simulink model "kopter_se_zavazim_LQR"  (R2024b)
settings: Solver=FixedStepAuto  StartTime=0.0  StopTime=30  FixedStep=0.01  RelTol=1e-3
values from neighbouring files (symbols this model uses):
  b_moment = 5.4e-6    (= 5.4e-06)    [parametry_kopter_se_zavazim.m]
  d = 1    [parametry_kopter_se_zavazim.m]
  g = 9.81    [parametry_kopter_se_zavazim.m]
  Ip = m*d^2    (= 1)    [parametry_kopter_se_zavazim.m]
  Ixx = 0.0222    [parametry_kopter_se_zavazim.m]
  Iyy = 0.0222    [parametry_kopter_se_zavazim.m]
  Izz = 0.0429    [parametry_kopter_se_zavazim.m]
  k_thrust = 2.3e-3    (= 0.0023)    [parametry_kopter_se_zavazim.m]
  ki_lqr = K_ex_lqr(:, 17:20)    [odvozeni_stavova_regulace_OTHER_ANGLES.m]
  kimot_lqr = Kmot_ex_lqr(:, 17:20)    [odvozeni_stavova_regulace_OTHER_ANGLES.m]
  kp_lqr = K_ex_lqr(:, 1:16)    [odvozeni_stavova_regulace_OTHER_ANGLES.m]
  kpmot_lqr = Kmot_ex_lqr(:, 1:16)    [odvozeni_stavova_regulace_OTHER_ANGLES.m]
  l = 0.2051    [parametry_kopter_se_zavazim.m]
  L_observer = place(Ac', Cc', poles_obs)'    [odvozeni_stavova_regulace_OTHER_ANGLES.m]
  M = 2    [parametry_kopter_se_zavazim.m]
  m = 1    [parametry_kopter_se_zavazim.m]
  Us_p = [(M+m)*g; 0; 0; 0]    [parametry_kopter_se_zavazim.m]
  Xinit_ss = [Xinit_matrix; [0 0 0 0 0 0 0 0]']    [parametry_kopter_se_zavazim.m]
  Xs_p = [0;0;0; 0;0;0; 0;0; 0;0;0; 0;0;0; 0;0]    [parametry_kopter_se_zavazim.m]
undefined symbols (not defined in the file or in its folder): L
libraries: simulink_extras x10
(part 3 of 3)

== matlab function kopter_se_zavazim_LQR/Nelinearni State-Space (se zavazim)_other_angles/A ==
  data: roll input; A output; pitch input; yaw input; alpha input; beta input; droll input; dpitch input; dyaw input; dalpha input; dbeta input; Ixx parameter; Iyy parameter; Izz parameter; M parameter; Ip parameter; d parameter; m parameter
function A = fcn(roll, pitch, yaw, alpha, beta, droll, dpitch, dyaw, dalpha, dbeta, Ixx, Iyy, Izz, M, Ip, d, m)
% Matice dynamiky A

phi_t = roll;
theta_t = pitch;
psi_t = yaw;

alpha_t = alpha;
beta_t = beta;

phi_dot_t = droll;
theta_dot_t = dpitch;
psi_dot_t = dyaw;

alpha_dot_t = dalpha;
beta_dot_t = dbeta;

A = [ 
0, 0, 0, 0, 0, 0, 0, 0, 1, 0, 0,                                                                                                                                                                                                                                                                                                                                                                                                                                                                                                           0,                                                                                                                                                                                                                                                                                                                                                                                                                                                                                                                                                                                                                                                                                                                              0,                                                                                                                                                                                            0,                                                          0,                                                  0;
0, 0, 0, 0, 0, 0, 0, 0, 0, 1, 0,                                                                                                                                                                                                                                                                                                                                                                                                                                                                                                           0,                                                                                                                                                                                                                                                                                                                                                                                                                                                                                                                                                                                                                                                                                                                              0,                                                                                                                                                                                            0,                                                          0,                                                  0;
0, 0, 0, 0, 0, 0, 0, 0, 0, 0, 1,                                                                                                                                                                                                                                                                                                                                                                                                                                                                                                           0,                                                                                                                                                                                                                                                                                                                                                                                                                                                                                                                                                                                                                                                                                                                              0,                                                                                                                                                                                            0,                                                          0,                                                  0;
0, 0, 0, 0, 0, 0, 0, 0, 0, 0, 0,                                                                                                                                                                                                                                                                                                                                                                                                                                                                                                           1,                                                                                                                                                                                                                                                                                                                                                                                                                                                                                                                                                                                                                                                                                                                              0,                                                                                                                                                                                            0,                                                          0,                                                  0;
0, 0, 0, 0, 0, 0, 0, 0, 0, 0, 0,                                                                                                                                                                                                                                                                                                                                                                                                                                                                                                           0,                                                                                                                                                                                                                                                                                                                                                                                                                                                                                                                                                                                                                                                                                                                              1,                                                                                                                                                                                            0,                                                          0,                                                  0;
0, 0, 0, 0, 0, 0, 0, 0, 0, 0, 0,                                                                                                                                                                                                                                                                                                                                                                                                                                                                                                           0,                                                                                                                                                                                                                                                                                                                                                                                                                                                                                                                                                                                                                                                                                                                              0,                                                                                                                                                                                            1,                                                          0,                                                  0;
0, 0, 0, 0, 0, 0, 0, 0, 0, 0, 0,                                                                                                                                                                                                                                                                                                                                                                                                                                                                                                           0,                                                                                                                                                                                                                                                                                                                                                                                                                                                                                                                                                                                                                                                                                                                              0,                                                                                                                                                                                            0,                                                          1,                                                  0;
0, 0, 0, 0, 0, 0, 0, 0, 0, 0, 0,                                                                                                                                                                                                                                                                                                                                                                                                                                                                                                           0,                                                                                                                                                                                                                                                                                                                                                                                                                                                                                                                                                                                                                                                                                                                              0,                                                                                                                                                                                            0,                                                          0,                                                  1;
0, 0, 0, 0, 0, 0, 0, 0, 0, 0, 0,                                                                                                                                                                                                                                                                                                                                                                                                                                                                                                           0,                                                                                                                                                                                                                                                                                                                                                                                                                                                                                                                                                                                                                                                                                                                              0,                                                                                                                                                                                            0,       (alpha_dot_t*d*m*cos(beta_t)^3*sin(alpha_t))/(M + m),  (beta_dot_t*d*m*cos(beta_t)*sin(alpha_t))/(M + m);
0, 0, 0, 0, 0, 0, 0, 0, 0, 0, 0,                                                                                                                                                                                                                                                                                                                                                                                                                                                                                                           0,                                                                                                                                                                                                                                                                                                                                                                                                                                                                                                                                                                                                                                                                                                                              0,                                                                                                                                                                                            0, -(alpha_dot_t*d*m*sin(beta_t)*(sin(beta_t)^2 - 1))/(M + m),               (beta_dot_t*d*m*sin(beta_t))/(M + m);
0, 0, 0, 0, 0, 0, 0, 0, 0, 0, 0,                                                                                                                                                                                                                                                                                                                                                                                                                                                                                                           0,                                                                                                                                                                                                                                                                                                                                                                                                                                                                                                                                                                                                                                                                                                                              0,                                                                                                                                                                                            0,      -(alpha_dot_t*d*m*cos(alpha_t)*cos(beta_t)^3)/(M + m), -(beta_dot_t*d*m*cos(alpha_t)*cos(beta_t))/(M + m);
0, 0, 0, 0, 0, 0, 0, 0, 0, 0, 0,                                       (sin(theta_t)*(Ixx*Izz*theta_dot_t - Izz^2*theta_dot_t + Iyy*Izz*theta_dot_t - Iyy^2*theta_dot_t*cos(phi_t)^2 + Izz^2*theta_dot_t*cos(phi_t)^2 + Ixx*Iyy*theta_dot_t*cos(phi_t)^2 - Ixx*Izz*theta_dot_t*cos(phi_t)^2 - Iyy^2*psi_dot_t*cos(phi_t)*cos(theta_t)*sin(phi_t) + Izz^2*psi_dot_t*cos(phi_t)*cos(theta_t)*sin(phi_t) + Ixx*Iyy*psi_dot_t*cos(phi_t)*cos(theta_t)*sin(phi_t) - Ixx*Izz*psi_dot_t*cos(phi_t)*cos(theta_t)*sin(phi_t)))/(Iyy*Izz*cos(theta_t)), - ((Iyy*Izz + Ixx*Iyy*sin(theta_t)^2 - Iyy*Izz*sin(theta_t)^2 - Ixx*Iyy*sin(phi_t)^2*sin(theta_t)^2 + Ixx*Izz*sin(phi_t)^2*sin(theta_t)^2)*((Izz*theta_dot_t*sin(2*phi_t))/2 - (Iyy*theta_dot_t*sin(2*phi_t))/2 + Ixx*psi_dot_t*cos(theta_t) - Iyy*psi_dot_t*cos(theta_t) + Izz*psi_dot_t*cos(theta_t) + 2*Iyy*psi_dot_t*cos(phi_t)^2*cos(theta_t) - 2*Izz*psi_dot_t*cos(phi_t)^2*cos(theta_t)))/(Ixx*Iyy*Izz*(sin(theta_t)^2 - 1)) - (sin(theta_t)^2*(Iyy - Iyy*sin(phi_t)^2 + Izz*sin(phi_t)^2)*((Iyy*theta_dot_t*sin(2*phi_t))/2 - (Izz*theta_dot_t*sin(2*phi_t))/2 - 2*Ixx*psi_dot_t*cos(theta_t) + 2*Izz*psi_dot_t*cos(phi_t)^2*cos(theta_t) + 2*Iyy*psi_dot_t*cos(theta_t)*sin(phi_t)^2))/(Iyy*Izz*(sin(theta_t)^2 - 1)), (psi_dot_t*sin(2*phi_t)*(Iyy - Izz)*(Ixx^2*cos(2*theta_t) - Ixx^2 + Ixx*Iyy + Ixx*Izz + Iyy*Izz - Ixx*Iyy*cos(2*theta_t) - Ixx*Izz*cos(2*theta_t) + Iyy*Izz*cos(2*theta_t)))/(4*Ixx*Iyy*Izz),                                                          0,                                                  0;
0, 0, 0, 0, 0, 0, 0, 0, 0, 0, 0, -(Izz^2*theta_dot_t*sin(2*phi_t) - Izz^2*psi_dot_t*cos(theta_t) - Iyy^2*theta_dot_t*sin(2*phi_t) - Iyy^2*psi_dot_t*cos(theta_t) + Ixx*Iyy*psi_dot_t*cos(theta_t) + Ixx*Izz*psi_dot_t*cos(theta_t) + 2*Iyy*Izz*psi_dot_t*cos(theta_t) + Iyy^2*psi_dot_t*cos(2*phi_t)*cos(theta_t) - Izz^2*psi_dot_t*cos(2*phi_t)*cos(theta_t) + Ixx*Iyy*theta_dot_t*sin(2*phi_t) - Ixx*Izz*theta_dot_t*sin(2*phi_t) - Ixx*Iyy*psi_dot_t*cos(2*phi_t)*cos(theta_t) + Ixx*Izz*psi_dot_t*cos(2*phi_t)*cos(theta_t))/(2*Iyy*Izz),                                                                                                                                                                                                                                                                                                                                                                                                                                                                                                                                                                                                                                        -(psi_dot_t*cos(phi_t)*sin(phi_t)*sin(theta_t)*(Iyy - Izz)*(Iyy - Ixx + Izz))/(Iyy*Izz),                           (psi_dot_t*sin(2*theta_t)*(Iyy^2*cos(2*phi_t) - Izz^2*cos(2*phi_t) - Iyy^2 - Izz^2 + Ixx*Iyy + Ixx*Izz - Ixx*Iyy*cos(2*phi_t) + Ixx*Izz*cos(2*phi_t)))/(4*Iyy*Izz),                                                          0,                                                  0;
0, 0, 0, 0, 0, 0, 0, 0, 0, 0, 0,                                            (Ixx*Iyy*theta_dot_t - Izz^2*theta_dot_t - Iyy^2*theta_dot_t + Ixx*Izz*theta_dot_t + 2*Iyy*Izz*theta_dot_t - Iyy^2*theta_dot_t*cos(2*phi_t) + Izz^2*theta_dot_t*cos(2*phi_t) - Iyy^2*psi_dot_t*sin(2*phi_t)*cos(theta_t) + Izz^2*psi_dot_t*sin(2*phi_t)*cos(theta_t) + Ixx*Iyy*theta_dot_t*cos(2*phi_t) - Ixx*Izz*theta_dot_t*cos(2*phi_t) + Ixx*Iyy*psi_dot_t*sin(2*phi_t)*cos(theta_t) - Ixx*Izz*psi_dot_t*sin(2*phi_t)*cos(theta_t))/(2*Iyy*Izz*cos(theta_t)),                                                                                                                                                                                                                                                                                                                                                                                                                                                                                                                                                                                                                  (psi_dot_t*sin(theta_t)*(Iyy - Iyy*sin(phi_t)^2 + Izz*sin(phi_t)^2)*(Iyy - Ixx + Izz))/(Iyy*Izz*cos(theta_t)),                                                                                                       (psi_dot_t*cos(phi_t)*sin(phi_t)*sin(theta_t)*(Iyy - Izz)*(Iyy - Ixx + Izz))/(Iyy*Izz),                                                          0,                                                  0;
0, 0, 0, 0, 0, 0, 0, 0, 0, 0, 0,                                                                                                                                                                                                                                                                                                                                                                                                                                                                                                           0,                                                                                                                                                                                                                                                                                                                                                                                                                                                                                                                                                                                                                                                                                                                              0,                                                                                                                                                                                            0,                     (2*beta_dot_t*sin(beta_t))/cos(beta_t),                                                  0;
0, 0, 0, 0, 0, 0, 0, 0, 0, 0, 0,                                                                                                                                                                                                                                                                                                                                                                                                                                                                                                           0,                                                                                                                                                                                                                                                                                                                                                                                                                                                                                                                                                                                                                                                                                                                              0,                                                                                                                                                                                            0,                             -(alpha_dot_t*sin(2*beta_t))/2,                                                  0];

== matlab function kopter_se_zavazim_LQR/Nelinearni State-Space (se zavazim)_other_angles/B ==
  data: roll input; B output; pitch input; yaw input; alpha input; beta input; M parameter; Ixx parameter; Iyy parameter; Izz parameter; Ip parameter; d parameter; m parameter
function B = fcn(roll, pitch, yaw, alpha, beta, M, Ixx, Iyy, Izz, Ip, d, m)
% Matice vstupu do soustavy kvadrokoptery se zavazim

phi_t = roll;
theta_t = pitch;
psi_t = yaw;

alpha_t = alpha;
beta_t = beta;

B = [ 
                                                                                                                                                                                                                                                                                                                                                                                                                                                                                                                                                                                   0,                                                                                                                                                                           0,                                                                        0,                                                                                          0;
                                                                                                                                                                                                                                                                                                                                                                                                                                                                                                                                                                                   0,                                                                                                                                                                           0,                                                                        0,                                                                                          0;
                                                                                                                                                                                                                                                                                                                                                                                                                                                                                                                                                                                   0,                                                                                                                                                                           0,                                                                        0,                                                                                          0;
                                                                                                                                                                                                                                                                                                                                                                                                                                                                                                                                                                                   0,                                                                                                                                                                           0,                                                                        0,                                                                                          0;
                                                                                                                                                                                                                                                                                                                                                                                                                                                                                                                                                                                   0,                                                                                                                                                                           0,                                                                        0,                                                                                          0;
                                                                                                                                                                                                                                                                                                                                                                                                                                                                                                                                                                                   0,                                                                                                                                                                           0,                                                                        0,                                                                                          0;
                                                                                                                                                                                                                                                                                                                                                                                                                                                                                                                                                                                   0,                                                                                                                                                                           0,                                                                        0,                                                                                          0;
                                                                                                                                                                                                                                                                                                                                                                                                                                                                                                                                                                                   0,                                                                                                                                                                           0,                                                                        0,                                                                                          0;
(M*sin(phi_t)*sin(psi_t) + m*sin(phi_t)*sin(psi_t) + M*cos(phi_t)*cos(psi_t)*sin(theta_t) + m*cos(phi_t)*cos(psi_t)*sin(theta_t) - m*cos(beta_t)^2*sin(phi_t)*sin(psi_t) - m*cos(beta_t)^2*cos(phi_t)*cos(psi_t)*sin(theta_t) + m*cos(alpha_t)^2*cos(beta_t)^2*sin(phi_t)*sin(psi_t) + m*cos(alpha_t)*cos(beta_t)^2*cos(phi_t)*sin(alpha_t)*cos(theta_t) + m*cos(alpha_t)^2*cos(beta_t)^2*cos(phi_t)*cos(psi_t)*sin(theta_t) + m*cos(beta_t)*cos(psi_t)*sin(alpha_t)*sin(beta_t)*sin(phi_t) - m*cos(beta_t)*cos(phi_t)*sin(alpha_t)*sin(beta_t)*sin(psi_t)*sin(theta_t))/(M*(M + m)),                                                                                                                                                                           0,                                                                        0,                                                                                          0;
                                                                                                                                                                                              -(M*cos(psi_t)*sin(phi_t) - M*cos(phi_t)*sin(psi_t)*sin(theta_t) + m*cos(beta_t)^2*cos(psi_t)*sin(phi_t) - m*cos(beta_t)^2*cos(phi_t)*sin(psi_t)*sin(theta_t) + m*cos(beta_t)*sin(alpha_t)*sin(beta_t)*sin(phi_t)*sin(psi_t) - m*cos(alpha_t)*cos(beta_t)*cos(phi_t)*sin(beta_t)*cos(theta_t) + m*cos(beta_t)*cos(phi_t)*cos(psi_t)*sin(alpha_t)*sin(beta_t)*sin(theta_t))/(M*(M + m)),                                                                                                                                                                           0,                                                                        0,                                                                                          0;
                                                                                                                                                            (M*cos(phi_t)*cos(theta_t) + m*cos(phi_t)*cos(theta_t) - m*cos(alpha_t)^2*cos(beta_t)^2*cos(phi_t)*cos(theta_t) + m*cos(alpha_t)*cos(beta_t)^2*sin(alpha_t)*sin(phi_t)*sin(psi_t) - m*cos(alpha_t)*cos(beta_t)*cos(psi_t)*sin(beta_t)*sin(phi_t) + m*cos(alpha_t)*cos(beta_t)^2*cos(phi_t)*cos(psi_t)*sin(alpha_t)*sin(theta_t) + m*cos(alpha_t)*cos(beta_t)*cos(phi_t)*sin(beta_t)*sin(psi_t)*sin(theta_t))/(M*(M + m)),                                                                                                                                                                           0,                                                                        0,                                                                                          0;
                                                                                                                                                                                                                                                                                                                                                                                                                                                                                                                                                                                   0, -(Iyy*Izz + Ixx*Iyy*sin(theta_t)^2 - Iyy*Izz*sin(theta_t)^2 - Ixx*Iyy*sin(phi_t)^2*sin(theta_t)^2 + Ixx*Izz*sin(phi_t)^2*sin(theta_t)^2)/(Ixx*Iyy*Izz*(sin(theta_t)^2 - 1)), -(cos(phi_t)*sin(phi_t)*sin(theta_t)*(Iyy - Izz))/(Iyy*Izz*cos(theta_t)), -(sin(theta_t)*(Iyy - Iyy*sin(phi_t)^2 + Izz*sin(phi_t)^2))/(Iyy*Izz*(sin(theta_t)^2 - 1));
                                                                                                                                                                                                                                                                                                                                                                                                                                                                                                                                                                                   0,                                                                                                    -(cos(phi_t)*sin(phi_t)*sin(theta_t)*(Iyy - Izz))/(Iyy*Izz*cos(theta_t)),                    (Izz + Iyy*sin(phi_t)^2 - Izz*sin(phi_t)^2)/(Iyy*Izz),                                       -(sin(2*phi_t)*(Iyy - Izz))/(2*Iyy*Izz*cos(theta_t));
                                                                                                                                                                                                                                                                                                                                                                                                                                                                                                                                                                                   0,                                                                                  -(sin(theta_t)*(Iyy - Iyy*sin(phi_t)^2 + Izz*sin(phi_t)^2))/(Iyy*Izz*(sin(theta_t)^2 - 1)),                     -(sin(2*phi_t)*(Iyy - Izz))/(2*Iyy*Izz*cos(theta_t)),                -(Iyy - Iyy*sin(phi_t)^2 + Izz*sin(phi_t)^2)/(Iyy*Izz*(sin(theta_t)^2 - 1));
                                                                                                                                                                                                                                                                                                                                                                                                                                    -(cos(phi_t)*sin(alpha_t)*cos(theta_t) + cos(alpha_t)*sin(phi_t)*sin(psi_t) + cos(alpha_t)*cos(phi_t)*cos(psi_t)*sin(theta_t))/(M*d*cos(beta_t)),                                                                                                                                                                           0,                                                                        0,                                                                                          0;
                                                                                                                                                                                                                                                                                                                        (cos(beta_t)*cos(psi_t)*sin(phi_t) - cos(alpha_t)*cos(phi_t)*sin(beta_t)*cos(theta_t) - cos(beta_t)*cos(phi_t)*sin(psi_t)*sin(theta_t) + sin(alpha_t)*sin(beta_t)*sin(phi_t)*sin(psi_t) + cos(phi_t)*cos(psi_t)*sin(alpha_t)*sin(beta_t)*sin(theta_t))/(M*d),                                                                                                                                                                           0,                                                                        0,                                                                                          0];

== matlab function kopter_se_zavazim_LQR/Nelinearni State-Space (se zavazim)_other_angles/BQ ==
  data: BQ output; g parameter
function BQ = fcn(g)
% Matice vstupu tihy
BQ = [0 0 0 0 0 0 0 0 0 0 -g 0 0 0 0 0]';

== matlab function kopter_se_zavazim_LQR/Nelinearni State-Space (se zavazim)_other_angles/MATLAB Function ==
  data: u output; m1 input; m2 input; m3 input; m4 input; k_thrust parameter; b_moment parameter; L parameter
function u = fcn(m1, m2, m3, m4, k_thrust, b_moment, L)

Thrust = k_thrust*(m1^2 + m2^2 + m3^2 + m4^2);
Tau_roll = L*k_thrust*(m1^2 + m4^2 - m2^2 - m3^2);
Tau_pitch = L*k_thrust*(m4^2 + m3^2 - m1^2 - m2^2);
Tau_yaw = b_moment*(m1^2 + m3^2 - m2^2 - m4^2);

u = [Thrust; Tau_roll; Tau_pitch; Tau_yaw];

== matlab function kopter_se_zavazim_LQR/Otacky rotoru ==
  data: u input; m1 output; m2 output; m3 output; m4 output; b_moment parameter; k_thrust parameter; l parameter
function [m1, m2, m3, m4]= fcn(u, b_moment, k_thrust, l)

T = u(1);
Tau_phi = u(2);
Tau_theta = u(3);
Tau_psi = u(4);

m1 = ( (Tau_phi*b_moment - Tau_theta*b_moment + l*T*b_moment + l*Tau_psi*k_thrust)/(4*l*b_moment*k_thrust));
m2 = ( (-Tau_theta*b_moment - Tau_phi*b_moment + l*T*b_moment - l*Tau_psi*k_thrust)/(4*l*b_moment*k_thrust));
m3 = ( (Tau_theta*b_moment - Tau_phi*b_moment + l*T*b_moment + l*Tau_psi*k_thrust)/(4*l*b_moment*k_thrust));
m4 = ( (Tau_phi*b_moment + Tau_theta*b_moment + l*T*b_moment - l*Tau_psi*k_thrust)/(4*l*b_moment*k_thrust));

== matlab function kopter_se_zavazim_LQR/Mezni naklon1 ==
  data: angles input; out output
function out = fcn(angles)

if all(angles<=85) && all(angles>=-85)
    out = 0;
else
    out = 1;
end

== matlab function kopter_se_zavazim_LQR/Linearni State-Space (se zavazim)_other_angles1/Ac ==
  data: g parameter; M parameter; Ac output; m parameter; Ip parameter; d parameter
function Ac = fcn(g, M, m, Ip, d)
% Matice Ac linearizovana kvadrokoptera+zavazi

Ac = [
0, 0, 0,                 0,                  0, 0,                  0,                  0, 1, 0, 0, 0, 0, 0, 0, 0;
0, 0, 0,                 0,                  0, 0,                  0,                  0, 0, 1, 0, 0, 0, 0, 0, 0;
0, 0, 0,                 0,                  0, 0,                  0,                  0, 0, 0, 1, 0, 0, 0, 0, 0;
0, 0, 0,                 0,                  0, 0,                  0,                  0, 0, 0, 0, 1, 0, 0, 0, 0;
0, 0, 0,                 0,                  0, 0,                  0,                  0, 0, 0, 0, 0, 1, 0, 0, 0;
0, 0, 0,                 0,                  0, 0,                  0,                  0, 0, 0, 0, 0, 0, 1, 0, 0;
0, 0, 0,                 0,                  0, 0,                  0,                  0, 0, 0, 0, 0, 0, 0, 1, 0;
0, 0, 0,                 0,                  0, 0,                  0,                  0, 0, 0, 0, 0, 0, 0, 0, 1;
0, 0, 0,                 0,      (g*(M + m))/M, 0,            (g*m)/M,                  0, 0, 0, 0, 0, 0, 0, 0, 0;
0, 0, 0,    -(g*(M + m))/M,                  0, 0,                  0,            (g*m)/M, 0, 0, 0, 0, 0, 0, 0, 0;
0, 0, 0,                 0,                  0, 0,                  0,                  0, 0, 0, 0, 0, 0, 0, 0, 0;
0, 0, 0,                 0,                  0, 0,                  0,                  0, 0, 0, 0, 0, 0, 0, 0, 0;
0, 0, 0,                 0,                  0, 0,                  0,                  0, 0, 0, 0, 0, 0, 0, 0, 0;
0, 0, 0,                 0,                  0, 0,                  0,                  0, 0, 0, 0, 0, 0, 0, 0, 0;
0, 0, 0,                 0, -(g*(M + m))/(M*d), 0, -(g*(M + m))/(M*d),                  0, 0, 0, 0, 0, 0, 0, 0, 0;
0, 0, 0, (g*(M + m))/(M*d),                  0, 0,                  0, -(g*(M + m))/(M*d), 0, 0, 0, 0, 0, 0, 0, 0];

== matlab function kopter_se_zavazim_LQR/Linearni State-Space (se zavazim)_other_angles/Ac ==
  data: g parameter; M parameter; Ac output; m parameter; Ip parameter; d parameter
function Ac = fcn(g, M, m, Ip, d)
% Matice Ac linearizovana kvadrokoptera+zavazi

Ac = [
0, 0, 0,                 0,                  0, 0,                  0,                  0, 1, 0, 0, 0, 0, 0, 0, 0;
0, 0, 0,                 0,                  0, 0,                  0,                  0, 0, 1, 0, 0, 0, 0, 0, 0;
0, 0, 0,                 0,                  0, 0,                  0,                  0, 0, 0, 1, 0, 0, 0, 0, 0;
0, 0, 0,                 0,                  0, 0,                  0,                  0, 0, 0, 0, 1, 0, 0, 0, 0;
0, 0, 0,                 0,                  0, 0,                  0,                  0, 0, 0, 0, 0, 1, 0, 0, 0;
0, 0, 0,                 0,                  0, 0,                  0,                  0, 0, 0, 0, 0, 0, 1, 0, 0;
0, 0, 0,                 0,                  0, 0,                  0,                  0, 0, 0, 0, 0, 0, 0, 1, 0;
0, 0, 0,                 0,                  0, 0,                  0,                  0, 0, 0, 0, 0, 0, 0, 0, 1;
0, 0, 0,                 0,      (g*(M + m))/M, 0,            (g*m)/M,                  0, 0, 0, 0, 0, 0, 0, 0, 0;
0, 0, 0,    -(g*(M + m))/M,                  0, 0,                  0,            (g*m)/M, 0, 0, 0, 0, 0, 0, 0, 0;
0, 0, 0,                 0,                  0, 0,                  0,                  0, 0, 0, 0, 0, 0, 0, 0, 0;
0, 0, 0,                 0,                  0, 0,                  0,                  0, 0, 0, 0, 0, 0, 0, 0, 0;
0, 0, 0,                 0,                  0, 0,                  0,                  0, 0, 0, 0, 0, 0, 0, 0, 0;
0, 0, 0,                 0,                  0, 0,                  0,                  0, 0, 0, 0, 0, 0, 0, 0, 0;
0, 0, 0,                 0, -(g*(M + m))/(M*d), 0, -(g*(M + m))/(M*d),                  0, 0, 0, 0, 0, 0, 0, 0, 0;
0, 0, 0, (g*(M + m))/(M*d),                  0, 0,                  0, -(g*(M + m))/(M*d), 0, 0, 0, 0, 0, 0, 0, 0];

== matlab function kopter_se_zavazim_LQR/Linearni State-Space (se zavazim)_other_angles/Bc ==
  data: M parameter; Bc output; Ixx parameter; Iyy parameter; Izz parameter; m parameter
function Bc = fcn(M, Ixx, Iyy, Izz, m)
% Matice Ac linearizovana

Bc = [
        0,     0,     0,     0;
        0,     0,     0,     0;
        0,     0,     0,     0;
        0,     0,     0,     0;
        0,     0,     0,     0;
        0,     0,     0,     0;
        0,     0,     0,     0;
        0,     0,     0,     0;
        0,     0,     0,     0;
        0,     0,     0,     0;
1/(M + m),     0,     0,     0;
        0, 1/Ixx,     0,     0;
        0,     0, 1/Iyy,     0;
        0,     0,     0, 1/Izz;
        0,     0,     0,     0;
        0,     0,     0,     0];

== matlab function kopter_se_zavazim_LQR/Linearni State-Space (se zavazim)_other_angles/MATLAB Function ==
  data: u output; m1 input; m2 input; m3 input; m4 input; k_thrust parameter; b_moment parameter; L parameter
function u = fcn(m1, m2, m3, m4, k_thrust, b_moment, L)

Thrust = k_thrust*(m1^2 + m2^2 + m3^2 + m4^2);
Tau_roll = L*k_thrust*(m1^2 + m4^2 - m2^2 - m3^2);
Tau_pitch = L*k_thrust*(m4^2 + m3^2 - m1^2 - m2^2);
Tau_yaw = b_moment*(m1^2 + m3^2 - m2^2 - m4^2);

u = [Thrust; Tau_roll; Tau_pitch; Tau_yaw];

== matlab function kopter_se_zavazim_LQR/Linearni State-Space (se zavazim)_other_angles1/Bc ==
  data: M parameter; Bc output; Ixx parameter; Iyy parameter; Izz parameter; m parameter
function Bc = fcn(M, Ixx, Iyy, Izz, m)
% Matice Ac linearizovana

Bc = [
        0,     0,     0,     0;
        0,     0,     0,     0;
        0,     0,     0,     0;
        0,     0,     0,     0;
        0,     0,     0,     0;
        0,     0,     0,     0;
        0,     0,     0,     0;
        0,     0,     0,     0;
        0,     0,     0,     0;
        0,     0,     0,     0;
1/(M + m),     0,     0,     0;
        0, 1/Ixx,     0,     0;
        0,     0, 1/Iyy,     0;
        0,     0,     0, 1/Izz;
        0,     0,     0,     0;
        0,     0,     0,     0];
